simulink model "single_engine_neural_narma_l2_learned_260120"  (R2018b)
settings: Solver=VariableStepAuto  StartTime=0.0  StopTime=10.0  RelTol=1e-3
libraries: neural x1
settings Model: Creator=Paweł Tymiński  LastModifiedBy=Paweł Tymiński

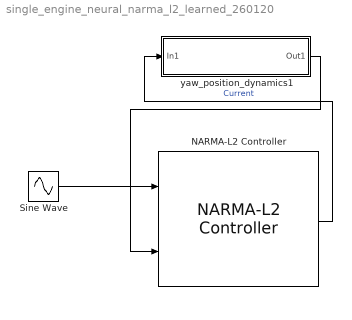
== system single_engine_neural_narma_l2_learned_260120 ==
  NARMA-L2 Controller : neural/Control Systems/NARMA-L2 Controller  Normalize=0  IW1_1=[-0.083112913336440649714;0.73363451470537821564]  IW3_2=[0.25660277370143558251;0.035307509884659700472]  IW5_3=1.4233621908085172247  LW2_1=[3.7785252021850115334 -1.2099415833116295982]  LW4_3=[-0.16448785742033977808 1.2361713858674965305]  LW5_4=-2.612118608866858871  LW6_5=1.4225418445046567051  LW6_2=-3.1195640877964763149  B1=[0.58852570745651089368;3.2215118520034473626]  B2=-0.79241928702528618977  B3=[1.2550802846057291795;-1.1496940107215367632]  B4=1.0944235532083537166  Limit_output=0  min_output=0  max_output=0  Use_Previous_Weights=1  Ts=0.001  S1=2  Ni=1  Nj=1  sim_file=0  trainfun=trainlm  Use_validation=1  Use_Testing=1  max_i=3  min_i=-3  max_i_int=0  min_i_int=0  sam_training=0  epochs=500  minp=-2.455060285275362908  maxp=2.495947464788551784  mint=-2.4550602852753495853  maxt=2.495947464788551784
      settings: SourceProductName=Neural Network Toolbox  SourceProductBaseCode=NN
  Sine Wave : Sin  SampleTime=0
  yaw_position_dynamics1 : Subsystem
  wires:
  Sine Wave/1 -> NARMA-L2 Controller/1
  NARMA-L2 Controller/1 -> yaw_position_dynamics1/1(In1)  "Current"
  yaw_position_dynamics1/1(Out1) -> NARMA-L2 Controller/2

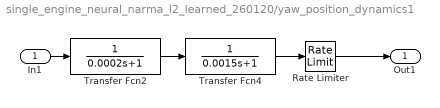
== system single_engine_neural_narma_l2_learned_260120/yaw_position_dynamics1 ==
  In1 : Inport
  Rate Limiter : RateLimiter  RisingSlewLimit=18.5  FallingSlewLimit=-18.5  SampleTimeMode=inherited
  Transfer Fcn2 : TransferFcn  Denominator=[0.0002 1]
  Transfer Fcn4 : TransferFcn  Denominator=[0.0015 1]
  Out1 : Outport
  wires:
  Transfer Fcn2/1 -> Transfer Fcn4/1
  In1/1 -> Transfer Fcn2/1
  Transfer Fcn4/1 -> Rate Limiter/1
  Rate Limiter/1 -> Out1/1
